simulink model "projetsi"  (R2021a)
settings: Solver=VariableStepAuto  StartTime=0.0  StopTime=10.0  RelTol=1e-3
libraries: aerolibanim x1
settings Model: Creator=Hp  LastModifiedBy=Hp

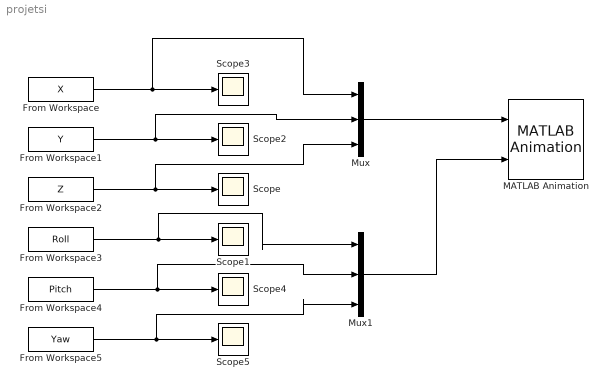
== system projetsi ==
  From Workspace : FromWorkspace  VariableName=X
  From Workspace1 : FromWorkspace  VariableName=Y
  From Workspace2 : FromWorkspace  VariableName=Z
  From Workspace3 : FromWorkspace  VariableName=Roll
  From Workspace4 : FromWorkspace  VariableName=Pitch
  From Workspace5 : FromWorkspace  VariableName=Yaw
  MATLAB Animation : aerolibanim/MATLAB Animation  Tag=Matlab Animation 6 DOF  Vehicles=1  Geometries='pa24-250_orange.ac'  BoundingBoxCoordinates=[-50,50,-50,50,-50,50]  CameraOffset=[-150,-50,0]  CameraViewAngle=4  SampleTime=0.01  FigurePosition=[1,41,1536,7.744000e+02]
      settings: SourceProductBaseCode=AE
  Mux : Mux  Inputs=3
  Mux1 : Mux  Inputs=3
  Scope{,1..5} (6 alike) : Scope
  wires:
  From Workspace/1 -> Mux/1, Scope3/1
  From Workspace1/1 -> Scope2/1, Mux/2
  From Workspace2/1 -> Mux/3, Scope/1
  From Workspace3/1 -> Mux1/1, Scope1/1
  From Workspace5/1 -> Mux1/3, Scope5/1
  Mux/1 -> MATLAB Animation/1
  Mux1/1 -> MATLAB Animation/2
  From Workspace4/1 -> Mux1/2, Scope4/1
